simulink model "abx_process"  (R2022b)
settings: Solver=VariableStepAuto  StartTime=0.0  StopTime=10.0  RelTol=1e-3
settings Model: Creator=Ranjeet  LastModifiedBy=Ranjeet
settings OptimizationCC: ReuseModelBlockBuffer=on

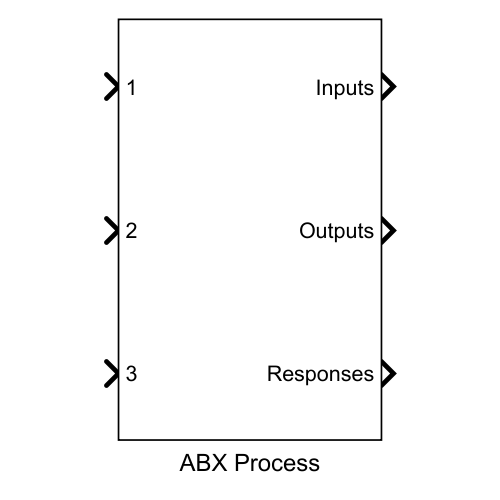
[thumbnail: Simulink's stored preview of the top-level diagram]
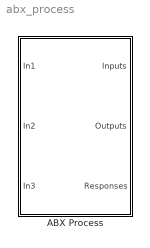
== system abx_process ==
  ABX Process : Subsystem

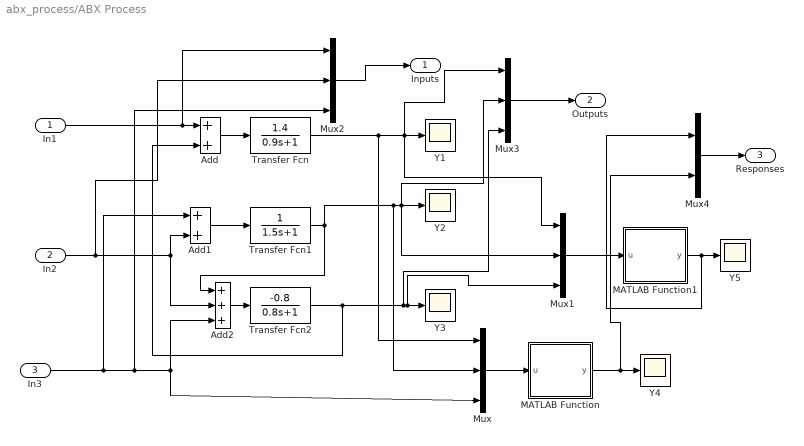
== system abx_process/ABX Process ==
  In1 : Inport
  In2 : Inport  Port=2
  In3 : Inport  Port=3
  Add : Sum
  Add1 : Sum
  Add2 : Sum  Inputs=+++
  MATLAB Function : MATLAB Function  TreatAsAtomicUnit=on
  MATLAB Function1 : MATLAB Function  TreatAsAtomicUnit=on
  Mux{,1..3} (4 alike) : Mux  Inputs=3
  Mux4 : Mux  Inputs=2
  Transfer Fcn : TransferFcn  Numerator=[1.4]  Denominator=[0.9 1]
  Transfer Fcn1 : TransferFcn  Denominator="[1.5  1]"
  Transfer Fcn2 : TransferFcn  Numerator=[-0.8]  Denominator=[0.8 1]
  Y{1..5} (5 alike) : Scope
  Inputs : Outport
  Outputs : Outport  Port=2
  Responses : Outport  Port=3
  wires:
  Transfer Fcn1/1 -> Mux/2, Mux3/2, Mux1/2, Y2/1, Add2/1
  Transfer Fcn2/1 -> Add/2, Mux3/3, Mux1/3, Y3/1
  In2/1 -> Mux2/2, Add1/2, Add2/2
  Transfer Fcn/1 -> Mux/1, Mux3/1, Mux1/1, Y1/1
  Add/1 -> Transfer Fcn/1
  Add2/1 -> Transfer Fcn2/1
  MATLAB Function1/1(y) -> Mux4/1, Y5/1
  Add1/1 -> Transfer Fcn1/1
  In1/1 -> Mux2/1, Add/1
  In3/1 -> Add1/1, Mux/3, Add2/3, Mux2/3
  Mux/1 -> MATLAB Function/1(u)
  Mux1/1 -> MATLAB Function1/1(u)
  MATLAB Function/1(y) -> Mux4/2, Y4/1
  Mux3/1 -> Outputs/1
  Mux4/1 -> Responses/1
  Mux2/1 -> Inputs/1

== matlab function abx_process/ABX Process/MATLAB Function ==
  data: u input; y output
function y = fcn(u)
%#codegen

y = 0.3 - 1.1*u(1) + 0.9*u(2) -0.6*u(3) - 0.1*(u(1)*u(2)*u(3));

== matlab function abx_process/ABX Process/MATLAB Function1 ==
  data: u input; y output
function y = fcn(u)
%#codegen

y = 1 + 2.1*u(1) + 1.7*u(2) - 1.9*u(3) - .5*(u(1)*u(2)*u(3));
